simulink model "ACMotorCL_Phi_cte"  (R2018b)
settings: Solver=ode23tb  StartTime=0.0  StopTime=10  RelTol=1e-3
InitFcn:
  | %f=50;
  | %VLLrms=400;
  | %Vph=VLLrms/sqrt(3);
  | %Irated=4000/(3*Vph);
  | %Vdrop_Stator= Irated*1.405;
  | 
  | %P=4000;
  | %Ws=4*pi*50/4; %Ws=4*pi*f/p (rad/s)
  | %Sr=(1500-1430)/1500;
  | %Wslip=Sr*Ws;
undefined symbols (not defined in the file): f
libraries: powerlib x14, simulink x4, powerlib_meascontrol x3
settings Model: Creator=Koosha  LastModifiedBy=Koosha

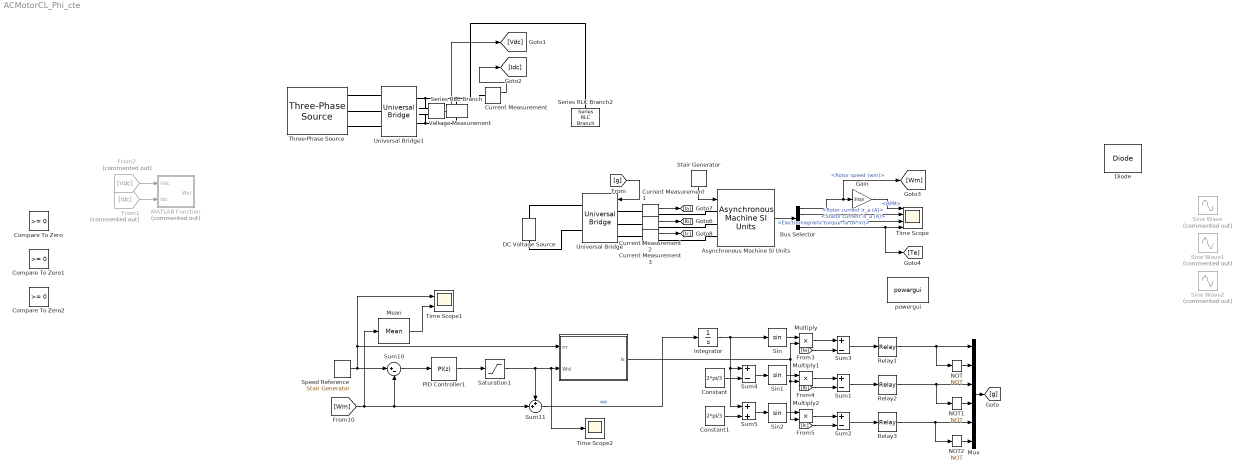
== system ACMotorCL_Phi_cte ==
  "  " : MATLAB Function  TreatAsAtomicUnit=on
  Asynchronous Machine SI Units : powerlib/Machines/Asynchronous Machine SI Units  RotorType=Squirrel-cage  PresetModel="15:  5.4 HP (4KW)   400 V  50Hz 1430 RPM"  MechanicalLoad=Torque Tm  ShowDetailedParameters=on  ReferenceFrame=Rotor  Units=SI  MeasurementBus=off  NominalParameters=[4000 400 50]  Stator=[1.405 0.005839]  Rotor=[1.395 0.005839]  Cage1=[0.4155 0.002066]  Cage2=[0.4168 0.0003495]  Lm=0.1722  Mechanical=[0.0131 0.002985 2]  PolePairs=2  InitialConditions=[1 0 0 0 0 0 0 0]  SimulateSaturation=off  Saturation=[14.03593122, 27.81365428, 53.79336849, 72.68890987, 97.98006896, 148.6815601, 215.7428561, 302.9841135, 428.7778367 ; 230, 322, 414, 460, 506, 552, 598, 644, 690]  LoadFlowParameters=1492000  TsPowergui=0  TsBlock=-1  IterativeModel=Trapezoidal non iterative  IterativeDiscreteModel=Trapezoidal non iterative  Pmec=1.492e+006
  Bus Selector : BusSelector  OutputSignals=Mechanical.Rotor speed (wm),Rotor measurements.Rotor current ir_a (A),Stator measurements.Stator current is_a (A),Mechanical.Electromagnetic torque Te (N*m)
  Compare To Zero : simulink/Logic and Bit Operations/Compare To Zero  relop=>=  OutDataTypeStr=boolean
  Compare To Zero1 : simulink/Logic and Bit Operations/Compare To Zero  relop=>=  OutDataTypeStr=boolean
  Compare To Zero2 : simulink/Logic and Bit Operations/Compare To Zero  relop=>=  OutDataTypeStr=boolean
  Constant : Constant  Value=2*pi/3
  Constant1 : Constant  Value=2*pi/3
  Current Measurement{,1..3} (4 alike) : powerlib/Measurements/Current Measurement  PhasorSimulation=off  OutputType=Complex  PSBequivalent=0
  DC Voltage Source : powerlib/Electrical Sources/DC Voltage Source  Amplitude=700  Measurements=None
  Diode : powerlib/Power Electronics/Diode  Ron=0.001  Lon=0  Vf=0.8  IC=0  UseSnubber=0  Rs=10  Cs=1e-9  Measurements=on
  From1 : From  Commented=on  GotoTag=Idc
  From2 : From  Commented=on  GotoTag=Vdc
  Gain : Gain  Gain=30/pi
  Integrator : Integrator
  MATLAB Function : MATLAB Function  Commented=on  TreatAsAtomicUnit=on
  Mean : powerlib_meascontrol/Measurements/Mean  Freq=60  Vinit=0  Ts=0
  Multiply : Product
  Multiply1 : Product
  Multiply2 : Product
  Mux : Mux  Inputs=6
  NOT : Logic  Operator=NOT  IconShape=distinctive  AllPortsSameDT=off  OutDataTypeStr=boolean
  NOT1 : Logic  Operator=NOT  IconShape=distinctive  AllPortsSameDT=off  OutDataTypeStr=boolean
  NOT2 : Logic  Operator=NOT  IconShape=distinctive  AllPortsSameDT=off  OutDataTypeStr=boolean
  PID Controller1 : simulink/Continuous/PID Controller  Controller=PI  Form=Parallel  TimeDomain=Discrete-time  SampleTime=-1  IntegratorMethod=Forward Euler  FilterMethod=Forward Euler  ControllerParametersSource=internal  P=2  I=25  D=1e-4  UseFilter=on  N=100  TunerSelectOption=Transfer Function Based (PID Tuner App)  InitialConditionSource=internal  InitialConditionForIntegrator=0  InitialConditionForFilter=0  DifferentiatorICPrevScaledInput=0  ExternalReset=none  TrackingMode=off  Kt=1  LimitOutput=off  UpperSaturationLimit=inf  LowerSaturationLimit=-inf  LinearizeAsGain=on  AntiWindupMode=none  Kb=1  POutMin=[]  POutMax=[]  IOutMin=[]  IOutMax=[]  DOutMin=[]  DOutMax=[]  NOutMin=[]  NOutMax=[]  SumOutMin=[]  SumOutMax=[]  SaturationOutMin=[]  SaturationOutMax=[]  PParamMin=[]  PParamMax=[]  IParamMin=[]  IParamMax=[]  DParamMin=[]  DParamMax=[]  NParamMin=[]  NParamMax=[]  KbParamMin=[]  KbParamMax=[]  KtParamMin=[]  KtParamMax=[]  KbOutMin=[]  KbOutMax=[]  KtOutMin=[]  KtOutMax=[]  IntegratorOutMin=[]  IntegratorOutMax=[]  FilterOutMin=[]  FilterOutMax=[]  SumI1OutMin=[]  SumI1OutMax=[]  SumI2OutMin=[]  SumI2OutMax=[]  SumI3OutMin=[]  SumI3OutMax=[]  SumI4OutMin=[]  SumI4OutMax=[]  SumDOutMin=[]  SumDOutMax=[]  DifferentiatorOutMin=[]  DifferentiatorOutMax=[]  FilterDiffOutCoefMin=[]  FilterDiffOutCoefMax=[]  ReciprocalOutMin=[]  ReciprocalOutMax=[]  SumDenOutMin=[]  SumDenOutMax=[]  SumNumOutMin=[]  SumNumOutMax=[]  DivideOutMin=[]  DivideOutMax=[]  IntegratorContinuousStateAttributes=''  IntegratorStateMustResolveToSignalObject=off  IntegratorRTWStateStorageClass=Auto  FilterContinuousStateAttributes=''  FilterStateMustResolveToSignalObject=off  FilterRTWStateStorageClass=Auto  ParallelPVariant=InternalParameters  IdealPVariant=Disabled  IVariant=InternalParameters  DVariant=Disabled  IntegratorVariant=Discrete  SatVariant=Disabled  AWVariant=Passthrough  PCopyVariant=Disabled  TRVariant=Disabled  FdbkBlocksVariant=Forward  IdealPFdbkVariant=Disabled  SatFdbkVariant=Disabled  DerivativeFilterVariant=Disabled  NVariant=Disabled  NCopyVariant=Disabled_SignalSpec  FilterICVariant=Disabled  IntegratorICVariant=InternalICs  ExternalResetVariant=Disabled  TRSumVariant=Passthrough  SumFdbkVariant=Disabled  SumVariant=Sum_PI
  Relay1 : Relay  OnSwitchValue=0.5  OffSwitchValue=-0.5  OutDataTypeStr=boolean
  Relay2 : Relay  OnSwitchValue=0.5  OffSwitchValue=-0.5  OutDataTypeStr=boolean
  Relay3 : Relay  OnSwitchValue=0.5  OffSwitchValue=-0.5  OutDataTypeStr=boolean
  Saturation1 : Saturate  UpperLimit=300  LowerLimit=-300
  Series RLC Branch : powerlib/Elements/Series RLC Branch  LConnTagsString=__new0  RConnTagsString=__new0  BranchType=C  Resistance=1  Inductance=1e-3  SetiL0=off  InitialCurrent=0  Capacitance=1e-6  Setx0=off  InitialVoltage=0  Measurements=None
  Series RLC Branch2 : powerlib/Elements/Series RLC Branch  LConnTagsString=__new0  RConnTagsString=__new0  BranchType=R  Resistance=1e-1  Inductance=1e-3  SetiL0=off  InitialCurrent=0  Capacitance=1e-6  Setx0=off  InitialVoltage=0  Measurements=None
  Sin : Trigonometry
  Sin1 : Trigonometry
  Sin2 : Trigonometry
  Sine Wave : Sin  Commented=on  Amplitude=0.85  Frequency=f*(2*pi)  SampleTime=0
  Sine Wave1 : Sin  Commented=on  Amplitude=0.85  Frequency=f*(2*pi)  Phase=-2*pi/3  SampleTime=0
  Sine Wave2 : Sin  Commented=on  Amplitude=0.85  Frequency=f*(2*pi)  Phase=2*pi/3  SampleTime=0
  Speed Reference : powerlib_meascontrol/Pulse & Signal Generators/Stair Generator  t=[0, 5]  e=[715*pi/30, 1430*pi/30]  Ts=0
      settings: SourceProductName=Simscape Power Systems
  Stair Generator : powerlib_meascontrol/Pulse & Signal Generators/Stair Generator  t=[0, 7]  e=[12, 24]  Ts=0
      settings: SourceProductName=Simscape Power Systems
  Sum1 : Sum  Inputs=+-  OutDataTypeStr=double
  Sum10 : Sum  Inputs=|+-
  Sum11 : Sum  Inputs=++|
  Sum2 : Sum  Inputs=+-  OutDataTypeStr=double
  Sum3 : Sum  Inputs=+-  OutDataTypeStr=double
  Sum4 : Sum  Inputs=+-
  Sum5 : Sum
  Three-Phase Source : powerlib/Electrical Sources/Three-Phase Source  InternalConnection=Yg  VoltagePhases=off  Voltage=700  PhaseAngle=0  Voltage_phases=[25e3 25e3 25e3]/sqrt(3)  PhaseAngles_phases=[0 -120 +120]  Frequency=50  NonIdealSource=off  SpecifyImpedance=off  Resistance=0.8929  Inductance=0  ShortCircuitLevel=100e6  BaseVoltage=0  XRratio=7  BusType=swing  Pref=10e3  Qref=0  Prefabc=[10e3, 10e3, 10e3]  Qrefabc=[0, 0, 0]  Qmin=-inf  Qmax=inf
  Time Scope : Scope  NumInputPorts=4
  Time Scope1 : Scope  NumInputPorts=2
  Time Scope2 : Scope
  Universal Bridge : powerlib/Power Electronics/Universal Bridge  Arms=3  SnubberResistance=10  SnubberCapacitance=1e-6  Device=IGBT / Diodes  Ron=1e-3  Lon=0  ForwardVoltages="[  0  0  ]"  ForwardVoltage=0  GTOparameters=[ 10e-6 , 20e-6 ]  IGBTparameters=[ 1e-6 , 2e-6 ]  Measurements=None  Measurements_2=None  converterType=Rectifier
  Universal Bridge1 : powerlib/Power Electronics/Universal Bridge  Arms=3  SnubberResistance=10  SnubberCapacitance=1e-6  Device=Diodes  Ron=1e-3  Lon=0  ForwardVoltages="[  0  0  ]"  ForwardVoltage=0  GTOparameters=[ 10e-6 , 20e-6 ]  IGBTparameters=[ 1e-6 , 2e-6 ]  Measurements=None  Measurements_2=None  converterType=Rectifier
  Voltage Measurement : powerlib/Measurements/Voltage Measurement  PhasorSimulation=off  OutputType=Complex  PSBequivalent=0
  powergui : powerlib/powergui  Priority=1  SimulationMode=Discrete  SampleTime=5e-6  frequency=60  Iterations=50  frequencyindice=50  Pbase=100e6  ErrMax=1e-4  UnitsV=kV  UnitsW=MW  buscounter=0  FunctionMessages=off  echomessages=off  EnableUseOfTLC=off  CurrentSourceSwitches=off  DisableSnubberDevices=off  DisableRonSwitches=off  DisableVfSwitches=off  DisplayEquations=off  SolverType=Tustin/Backward Euler (TBE)  Interpol=off  ExternalGateDelay=off  methode=off  Ts=100  x0status=blocks  SPID=off  SwTol=0  HookPort=off  RestoreLinks=warning  ResistiveCurrentMeasurement=off  Frange=[0:2:500]  Ylog=off  Xlog=on  ShowGrid=off  save=off  variable=ZData  structure=0  ZoomFFT=off  StartTime=0.0  cycles=1  DisplayStyle=1  fundamental=60  FreqAxis=off  MaxFrequency=1000  frequencyindicesteady=1  RmsSteady=1  display=off
  wires:
  Stair Generator/1 -> Asynchronous Machine SI Units/1
  Gain/1 -> Time Scope/1  "<RPM>"
  Asynchronous Machine SI Units/1 -> Bus Selector/1
  Bus Selector/1 -> [Wm], Gain/1  "<Rotor speed (wm)>"
  Relay1/1 -> Mux/1, NOT/1
  NOT/1 -> Mux/2
  Relay2/1 -> Mux/3, NOT1/1
  NOT1/1 -> Mux/4
  Relay3/1 -> Mux/5, NOT2/1
  NOT2/1 -> Mux/6
  Mux/1 -> [g]
  [g] -> Universal Bridge/1
  Sum5/1 -> Sin2/1
  Sum4/1 -> Sin1/1
  Constant1/1 -> Sum5/2
  Constant/1 -> Sum4/2
  Integrator/1 -> Sum5/1, Sum4/1, Sin/1
  Sum11/1 -> Integrator/1  "we"
  Multiply/1 -> Sum3/1
  Sin/1 -> Multiply/1
  Sin1/1 -> Multiply1/1
  Multiply1/1 -> Sum1/1
  Sin2/1 -> Multiply2/1
  Multiply2/1 -> Sum2/1
  "  "/1(Is) -> Multiply2/2, Multiply1/2, Multiply/2
  Bus Selector/2 -> Time Scope/2  "<Rotor current ir_a (A)>"
  Bus Selector/3 -> Time Scope/3  "<Stator current is_a (A)>"
  Bus Selector/4 -> [Te], Time Scope/4  "<Electromagnetic torque Te (N*m)>"
  From2/1 -> MATLAB Function/1(Vdc)
  From1/1 -> MATLAB Function/2(Idc)
  PID Controller1/1 -> Saturation1/1
  Speed Reference/1 -> Sum10/1, "  "/1(nr), Time Scope1/1
  [Wm] -> Mean/1, Sum10/2, Sum11/2
  Sum10/1 -> PID Controller1/1
  Current Measurement3/1 -> [Ic]
  Current Measurement2/1 -> [Ib]
  Current Measurement1/1 -> [Ia]
  Sum3/1 -> Relay1/1
  Sum1/1 -> Relay2/1
  Sum2/1 -> Relay3/1
  [Ia] -> Sum3/2
  [Ib] -> Sum1/2
  [Ic] -> Sum2/2
  Current Measurement/1 -> [Idc]
  Voltage Measurement/1 -> [Vdc]
  Saturation1/1 -> Time Scope2/1, "  "/2(Wsl), Sum11/1
  Mean/1 -> Time Scope1/2
  connections:
  Current Measurement2/LConn1 -- Universal Bridge/LConn2
  Universal Bridge/LConn3 -- Current Measurement3/LConn1
  Universal Bridge/LConn1 -- Current Measurement1/LConn1
  Current Measurement1/RConn1 -- Asynchronous Machine SI Units/LConn1
  Current Measurement2/RConn1 -- Asynchronous Machine SI Units/LConn2
  Current Measurement3/RConn1 -- Asynchronous Machine SI Units/LConn3
  Voltage Measurement/LConn2 -- Universal Bridge1/RConn2 -- Series RLC Branch/RConn1
  Series RLC Branch2/LConn1 -- Current Measurement/LConn1 -- Series RLC Branch/LConn1 -- Voltage Measurement/LConn1 -- Universal Bridge1/RConn1
  Universal Bridge1/LConn1 -- Three-Phase Source/RConn1
  Universal Bridge1/LConn3 -- Three-Phase Source/RConn3
  Universal Bridge1/LConn2 -- Three-Phase Source/RConn2
  DC Voltage Source/RConn1 -- Universal Bridge/RConn1
  DC Voltage Source/LConn1 -- Universal Bridge/RConn2

== matlab function ACMotorCL_Phi_cte/MATLAB Function ==
  data: Vdc input; Wsl output; Idc input
function Wsl = fcn(Vdc, Idc)
P=4000;
Ws=4*pi*50/4; %Ws=4*pi*f/p (rad/s)
Sr=(1500-1430)/1500;
Wslip=Sr*Ws;
Pva=Vdc*Idc;
Wsl=(Pva/P)*Wslip;
if Wsl > Wslip
    Wsl=Wslip;
end
end

== matlab function ACMotorCL_Phi_cte/   ==
  data: nr input; Wsl input; Is output
function Is = fcn(nr,Wsl)

f=(nr*30/pi)*4/120;
ws=1500*pi/30;
Lm=0.1722;
Rr=1.395;
Llr=0.005839;
Lr=Llr+Lm;
Tr=Lr/Rr;
Sigmar=Llr/Lm;


   Im=(400/sqrt(3))/(2*pi*f*Lm);
   Is=abs((1i*Wsl*Tr+1)/(1i*Wsl*(Sigmar/(1+Sigmar))*Tr+1))*Im;

end
